simulink model "sl_demo_16a"  (R2016a)
settings: Solver=VariableStepAuto  SolverMode=SingleTasking  StartTime=0.0  StopTime=dt*500  RelTol=1e-3
values from neighbouring files (symbols this model uses):
  dt = 0.05    [demo_double_integ.m]    (also in double_integ_env.m)
  dx0 = xold(2)    [demo_double_integ.m]
  x0 = xold(1)    [demo_double_integ.m]
settings Model: Creator=Yuri  LastModifiedBy=yjiang
settings DataIOCC: SaveFormat=Array  SaveState=on
settings DebuggingCC: SFUnexpectedBacktrackingDiag=error  SFNoUnconditionalDefaultTransitionDiag=error
settings GRTTargetCC: TargetLangStandard=C99 (ISO)  GeneratePreprocessorConditionals=Use local settings
settings ConfigComp: CovMetricSettings=dwe  CovHtmlReporting=off  CovSaveCumulativeToWorkspaceVar=off  CovSaveSingleToWorkspaceVar=off  CovExternalEMLEnable=on

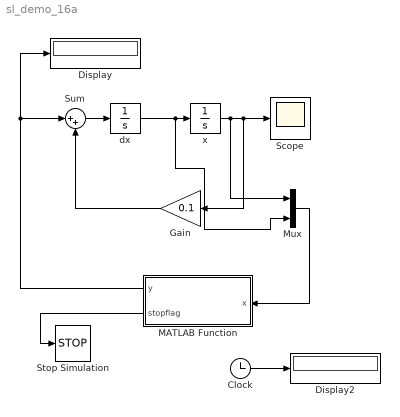
== system sl_demo_16a ==
  Clock : Clock
  Display : Display
  Display2 : Display
  Gain : Gain  Gain=0.1
  MATLAB Function : MATLAB Function  TreatAsAtomicUnit=on  SystemSampleTime=dt
      settings: PermitHierarchicalResolution=ParametersOnly
  Mux : Mux  Inputs=2
  Scope : Scope
  Stop Simulation : Stop
  Sum : Sum  Inputs=|++
  dx : Integrator  InitialCondition=dx0
  x : Integrator  InitialCondition=x0
  wires:
  dx/1 -> Mux/2, x/1
  MATLAB Function/1(y) -> Sum/1, Display/1
  x/1 -> Mux/1, Scope/1, Gain/1
  Sum/1 -> dx/1
  Gain/1 -> Sum/2
  Mux/1 -> MATLAB Function/1(x)
  MATLAB Function/2(stopflag) -> Stop Simulation/1
  Clock/1 -> Display2/1

== matlab function sl_demo_16a/MATLAB Function ==
  data: x input; y output double size=1; stopflag output
function [y, stopflag] = fcn(x)
%#codegen
y = 0;
stopflag = false;


coder.extrinsic('evalin');
coder.extrinsic('assignin');


%% compute new reward
if max(x) > 1 || min(x) <-1
    stopflag = true;
    r = -1000;
else
    r = 1/(100*x(1)^2+x(2)^2+0.01);
end

assignin('base', 'r', r);
assignin('base', 'x', x);                   %update new x
evalin('base', 'qt.update(xold, a, x, r);');
evalin('base', 'xold = x;');
evalin('base', 'a = qt.getAction(x);');     %get new action

y = evalin('base', 'a');
